simulink model "BPSK"  (R2021a)
settings: Solver=VariableStepAuto  StartTime=0.0  StopTime=10.0  RelTol=1e-3
libraries: commrandsrc3 x1
settings Model: Creator=Dell  LastModifiedBy=Dell

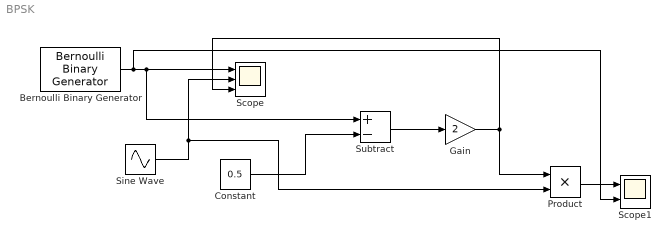
== system BPSK ==
  Bernoulli Binary Generator : commrandsrc3/Bernoulli Binary Generator  ProbabilityOfZero=0.5  SeedSource=Auto  Seed=0  SampleTime=2  SamplesPerFrame=1  OutputDataType=double  SimulateUsing=Interpreted execution
  Constant : Constant  Value=0.5
  Gain : Gain  Gain=2
  Product : Product
  Scope : Scope  NumInputPorts=3
  Scope1 : Scope  NumInputPorts=2
  Sine Wave : Sin  Frequency=4*pi  SampleTime=1/3200*pi
  Subtract : Sum  Inputs=+-
  wires:
  Constant/1 -> Subtract/2
  Subtract/1 -> Gain/1
  Gain/1 -> Product/1, Scope/3
  Sine Wave/1 -> Product/2, Scope/2
  Product/1 -> Scope1/1
  Bernoulli Binary Generator/1 -> Scope/1, Subtract/1, Scope1/2
